simulink model "ex4_custo"  (R2020b)
settings: Solver=VariableStepAuto  StartTime=0.0  StopTime=10.0  RelTol=1e-3
values from neighbouring files (symbols this model uses):
  h = 1    [ex4_custo_script.m]
  x0 = [1;1]    [ex4_custo_script.m]
undefined symbols (not defined in the file or in its folder): F_ARE
settings Model: Creator=lucas  LastModifiedBy=lucas

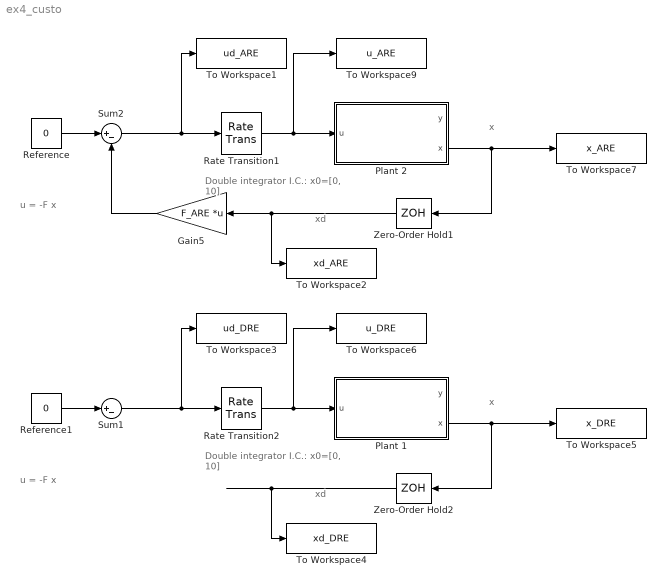
== system ex4_custo ==
  note: Double integrator
      | I.C.: x0=[0, 10]
  note: u = -F x
  note: x
  note: xd
  note: Double integrator
      | I.C.: x0=[0, 10]
  note: u = -F x
  note: x
  note: xd
  Gain5 : Gain  Gain=F_ARE  Multiplication=Matrix(K*u)
  Plant 1 : Subsystem
      mask Display:
      | text(.5,.6,'dx/dt = Ax + Bu','horizontalAlignment', 'center','verticalAlignment', 'middle','texmode','on')
      | text(.5,.4,'y = Cx + Du','horizontalAlignment', 'center','verticalAlignment', 'middle','texmode','on')
      | port_label('input',1,'u')
      | port_label('output',1,'y')
      | port_label('output',2,'x')
  Plant 2 : Subsystem
      mask Display:
      | text(.5,.6,'dx/dt = Ax + Bu','horizontalAlignment', 'center','verticalAlignment', 'middle','texmode','on')
      | text(.5,.4,'y = Cx + Du','horizontalAlignment', 'center','verticalAlignment', 'middle','texmode','on')
      | port_label('input',1,'u')
      | port_label('output',1,'y')
      | port_label('output',2,'x')
  Rate Transition1 : RateTransition  Integrity=off  OutPortSampleTime=h
  Rate Transition2 : RateTransition  Integrity=off  OutPortSampleTime=h
  Reference : Constant  Value=0  SampleTime=h
  Reference1 : Constant  Value=0  SampleTime=h
  Sum1 : Sum  Inputs=|+-
  Sum2 : Sum  Inputs=|+-
  To Workspace1 : ToWorkspace  VariableName=ud_ARE  SaveFormat=Timeseries  SampleTime=-1
  To Workspace2 : ToWorkspace  VariableName=xd_ARE  SaveFormat=Timeseries  SampleTime=-1
  To Workspace3 : ToWorkspace  VariableName=ud_DRE  SaveFormat=Timeseries  SampleTime=-1
  To Workspace4 : ToWorkspace  VariableName=xd_DRE  SaveFormat=Timeseries  SampleTime=-1
  To Workspace5 : ToWorkspace  VariableName=x_DRE  SaveFormat=Timeseries  SampleTime=-1
  To Workspace6 : ToWorkspace  VariableName=u_DRE  SaveFormat=Timeseries  SampleTime=-1
  To Workspace7 : ToWorkspace  VariableName=x_ARE  SaveFormat=Timeseries  SampleTime=-1
  To Workspace9 : ToWorkspace  VariableName=u_ARE  SaveFormat=Timeseries  SampleTime=-1
  Zero-Order Hold1 : ZeroOrderHold  SampleTime=h
  Zero-Order Hold2 : ZeroOrderHold  SampleTime=h
  wires:
  Reference/1 -> Sum2/1
  Sum2/1 -> To Workspace1/1, Rate Transition1/1
  Zero-Order Hold1/1 -> To Workspace2/1, Gain5/1
  Plant 2/2(x) -> To Workspace7/1, Zero-Order Hold1/1
  Gain5/1 -> Sum2/2
  Rate Transition1/1 -> Plant 2/1(u), To Workspace9/1
  Sum1/1 -> To Workspace3/1, Rate Transition2/1
  Plant 1/2(x) -> To Workspace5/1, Zero-Order Hold2/1
  Reference1/1 -> Sum1/1
  Zero-Order Hold2/1 -> To Workspace4/1
  Rate Transition2/1 -> Plant 1/1(u), To Workspace6/1
  ? -> Sum1/2

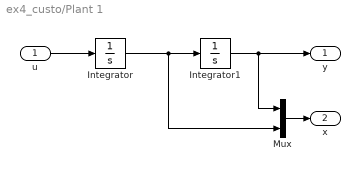
== system ex4_custo/Plant 1 ==
  u : Inport
  Integrator : Integrator  InitialCondition=x0(2)
  Integrator1 : Integrator  InitialCondition=x0(1)
  Mux : Mux  Inputs=2
  y : Outport
  x : Outport  Port=2
  wires:
  Integrator/1 -> Mux/2, Integrator1/1
  Integrator1/1 -> Mux/1, y/1
  u/1 -> Integrator/1
  Mux/1 -> x/1

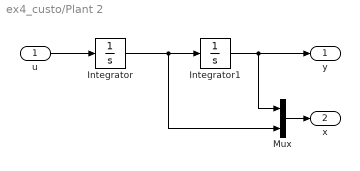
== system ex4_custo/Plant 2 ==
  u : Inport
  Integrator : Integrator  InitialCondition=x0(2)
  Integrator1 : Integrator  InitialCondition=x0(1)
  Mux : Mux  Inputs=2
  y : Outport
  x : Outport  Port=2
  wires:
  Integrator/1 -> Mux/2, Integrator1/1
  Integrator1/1 -> Mux/1, y/1
  u/1 -> Integrator/1
  Mux/1 -> x/1
